simulink model "DC_H_Bridge_LC_Oscillation_MOSFET"  (R2022b)
settings: Solver=VariableStepAuto  StartTime=0.0  StopTime=10  RelTol=1e-3
libraries: spsIGBTLib x4, spsMosfetLib x4, spsSeriesRLCBranchLib x3, spsVoltageMeasurementLib x3, spsDCVoltageSourceLib x2, simulink x1, spsSawtoothGeneratorLib x1, spspowerguiLib x1
settings Model: Creator=SIDDHARTH  LastModifiedBy=SIDDHARTH

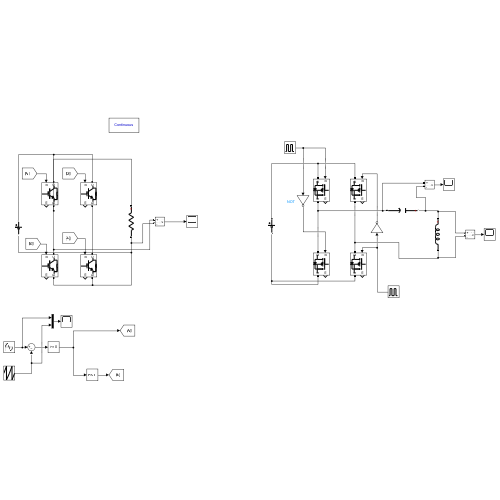
[thumbnail: Simulink's stored preview of the top-level diagram]
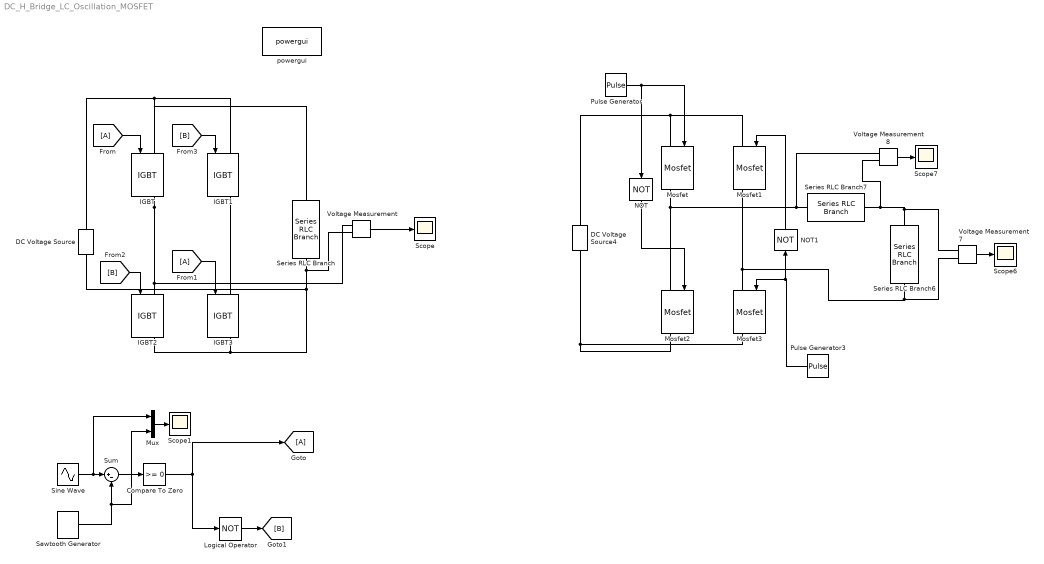
== system DC_H_Bridge_LC_Oscillation_MOSFET ==
  Compare To Zero : simulink/Logic and Bit Operations/Compare To Zero  relop=>=  OutDataTypeStr=boolean
  DC Voltage Source : spsDCVoltageSourceLib/DC Voltage Source  Amplitude=100  Measurements=None
  DC Voltage Source4 : spsDCVoltageSourceLib/DC Voltage Source  Amplitude=24  Measurements=None
  From : From
  From1 : From
  Goto : Goto
  IGBT{,1..3} (4 alike) : spsIGBTLib/IGBT  Ron=0.001  Lon=0  Vf=1  Tf=1e-6  Tt=2e-6  IC=0  Rs=1e5  Cs=inf  Measurements=on
  Logical Operator : Logic  Operator=NOT  AllPortsSameDT=off  OutDataTypeStr=boolean
  Mosfet{,1..3} (4 alike) : spsMosfetLib/Mosfet  Ron=0.1  Lon=0  Rd=0.01  Vfd=0  IC=0  Rs=1e5  Cs=inf  Measurements=on
  Mux : Mux  Inputs=2
  NOT : Logic  Operator=NOT  IconShape=distinctive  AllPortsSameDT=off  OutDataTypeStr=boolean
  NOT1 : Logic  Operator=NOT  IconShape=distinctive  AllPortsSameDT=off  OutDataTypeStr=boolean
  Pulse Generator : DiscretePulseGenerator  PulseType=Time based  Period=1/50000  PulseWidth=75
  Pulse Generator3 : DiscretePulseGenerator  PulseType=Time based  Period=1/50000  PulseWidth=75
  Sawtooth Generator : spsSawtoothGeneratorLib/Sawtooth Generator  Freq=1e3  Phase=180  Ts=0
  Scope{,1,6..7} (4 alike) : Scope
  Series RLC Branch : spsSeriesRLCBranchLib/Series RLC Branch  LConnTagsString=__new0  RConnTagsString=__new0  BranchType=R  Resistance=10  Inductance=1e-3  SetiL0=off  InitialCurrent=0  Capacitance=1e-6  Setx0=off  InitialVoltage=0  Measurements=None
  Series RLC Branch6 : spsSeriesRLCBranchLib/Series RLC Branch  LConnTagsString=__new0  RConnTagsString=__new0  BranchType=L  Resistance=10  Inductance=1/(4*pi*pi*50000*(100e-6))  SetiL0=off  InitialCurrent=0  Capacitance=1e-6  Setx0=off  InitialVoltage=0  Measurements=None
  Series RLC Branch7 : spsSeriesRLCBranchLib/Series RLC Branch  LConnTagsString=__new0  RConnTagsString=__new0  BranchType=C  Resistance=10  Inductance=1.02  SetiL0=off  InitialCurrent=0  Capacitance=100e-6  Setx0=off  InitialVoltage=0  Measurements=None
  Sine Wave : Sin  Amplitude=0.9  Frequency=50  SampleTime=0
  Sum : Sum  Inputs=|+-
  Voltage Measurement : spsVoltageMeasurementLib/Voltage Measurement  PhasorSimulation=off  OutputType=Complex  PSBequivalent=0
  Voltage Measurement7 : spsVoltageMeasurementLib/Voltage Measurement  PhasorSimulation=off  OutputType=Complex  PSBequivalent=0
  Voltage Measurement8 : spsVoltageMeasurementLib/Voltage Measurement  PhasorSimulation=off  OutputType=Complex  PSBequivalent=0
  powergui : spspowerguiLib/powergui  Priority=1  SimulationMode=Continuous  SampleTime=50e-6  frequency=60  Iterations=50  frequencyindice=0  Pbase=100e6  ErrMax=1e-4  UnitsV=kV  UnitsW=MW  buscounter=0  FunctionMessages=off  echomessages=off  EnableUseOfTLC=off  CurrentSourceSwitches=off  DisableSnubberDevices=off  DisableRonSwitches=off  DisableVfSwitches=off  DisplayEquations=off  AutomaticDiscreteSolvers=off  SolverType=Tustin/Backward Euler (TBE)  Interpol=off  ExternalGateDelay=off  methode=off  Ts=100  x0status=blocks  SPID=on  SwTol=0  HookPort=off  NonlinearTolerance=1e-4  nMaxIteration=100  ContinueOnMaxIteration=off  RestoreLinks=warning  ResistiveCurrentMeasurement=off  Frange=[0:2:500]  Ylog=off  Xlog=on  ShowGrid=off  save=off  variable=ZData  structure=0  ZoomFFT=off  StartTime=0.0  cycles=1  DisplayStyle=1  fundamental=60  FreqAxis=off  MaxFrequency=1000  frequencyindicesteady=1  RmsSteady=1  display=off
  wires:
  [B] -> IGBT2/1
  Voltage Measurement/1 -> Scope/1
  [B] -> IGBT1/1
  Compare To Zero/1 -> Goto/1, Logical Operator/1
  From1/1 -> IGBT3/1
  Sine Wave/1 -> Mux/1, Sum/1
  Mux/1 -> Scope1/1
  Sum/1 -> Compare To Zero/1
  From/1 -> IGBT/1
  Sawtooth Generator/1 -> Mux/2, Sum/2
  Logical Operator/1 -> [B]
  Pulse Generator/1 -> Mosfet/1, NOT/1
  Pulse Generator3/1 -> NOT1/1, Mosfet3/1
  Voltage Measurement7/1 -> Scope6/1
  NOT/1 -> Mosfet2/1
  NOT1/1 -> Mosfet1/1
  Voltage Measurement8/1 -> Scope7/1
  connections:
  IGBT/LConn1 -- IGBT1/LConn1 -- DC Voltage Source/RConn1
  IGBT2/LConn1 -- IGBT/RConn1 -- Series RLC Branch/LConn1 -- Voltage Measurement/LConn1
  IGBT2/RConn1 -- Series RLC Branch/RConn1 -- Voltage Measurement/LConn2 -- DC Voltage Source/LConn1 -- IGBT3/RConn1
  IGBT1/RConn1 -- IGBT3/LConn1
  Mosfet/RConn1 -- Voltage Measurement8/LConn1 -- Series RLC Branch7/RConn1 -- Mosfet2/LConn1
  Mosfet1/RConn1 -- Voltage Measurement7/LConn2 -- Series RLC Branch6/RConn1 -- Mosfet3/LConn1
  Mosfet/LConn1 -- Mosfet1/LConn1 -- DC Voltage Source4/RConn1
  Mosfet2/RConn1 -- DC Voltage Source4/LConn1 -- Mosfet3/RConn1
  Series RLC Branch6/LConn1 -- Voltage Measurement7/LConn1 -- Voltage Measurement8/LConn2 -- Series RLC Branch7/LConn1
